simulink model "ysw3_40"  (R2014a)
settings: Solver=ode45  StartTime=0.0  StopTime=10.0  RelTol=1e-3
settings Model: Creator=Administrator  LastModifiedBy=Administrator

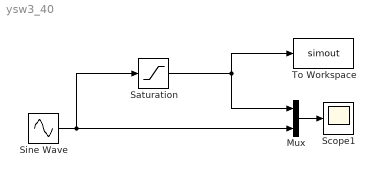
== system ysw3_40 ==
  Mux : Mux  Inputs=2
  Saturation : Saturate
  Scope1 : Scope
      settings: TimeRange=10
  Sine Wave : Sin  SampleTime=0.1
  To Workspace : ToWorkspace  VariableName=simout  SaveFormat=Timeseries  SampleTime=-1
  wires:
  Mux/1 -> Scope1/1
  Sine Wave/1 -> Saturation/1, Mux/2
  Saturation/1 -> Mux/1, To Workspace/1
